simulink model "PSO_tunning_PID"  (R2017a)
settings: Solver=ode23s  StartTime=0.0  StopTime=10  RelTol=1000000
undefined symbols (not defined in the file or in its folder): kk
libraries: simulink x2
settings Model: Creator=abdul  LastModifiedBy=Dr. Javed
settings DataIOCC: SaveFormat=Array

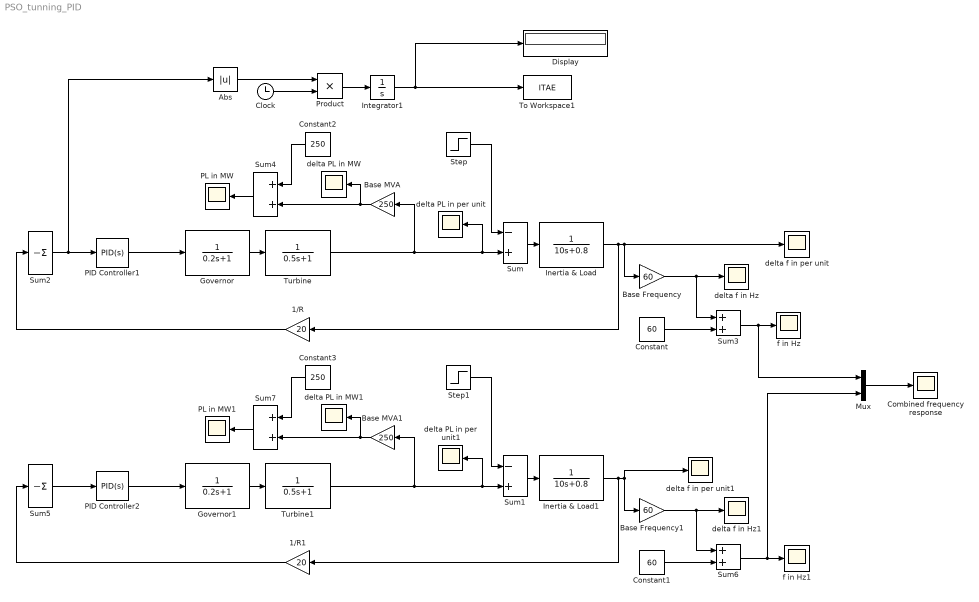
== system PSO_tunning_PID ==
  1/R : Gain  Gain=20
  1/R1 : Gain  Gain=20
  Abs : Abs
  Base Frequency : Gain  Gain=60
  Base Frequency1 : Gain  Gain=60
  Base MVA : Gain  Gain=250
  Base MVA1 : Gain  Gain=250
  Clock : Clock
  "Combined frequency response " : Scope
  Constant : Constant  Value=60
  Constant1 : Constant  Value=60
  Constant2 : Constant  Value=250
  Constant3 : Constant  Value=250
  Display : Display
      settings: Format=decimal (Stored Integer)
  Governor : TransferFcn  Denominator=[0.2 1]
  Governor1 : TransferFcn  Denominator=[0.2 1]
  Inertia & Load : TransferFcn  Denominator=[10 0.8]
  Inertia & Load1 : TransferFcn  Denominator=[10 0.8]
  Integrator1 : Integrator
  Mux : Mux  Inputs=2
  PID Controller1 : simulink/Continuous/PID Controller  Controller=PID  TimeDomain=Continuous-time  SampleTime=-1  IntegratorMethod=Forward Euler  FilterMethod=Forward Euler  Form=Parallel  UseFilter=on  ControllerParametersSource=internal  P=kk(1)  I=kk(2)  D=kk(3)  N=100  InitialConditionSource=internal  InitialConditionForIntegrator=0  InitialConditionForFilter=0  ExternalReset=none  LimitOutput=off  UpperSaturationLimit=inf  LowerSaturationLimit=-inf  LinearizeAsGain=on  AntiWindupMode=none  Kb=1  TrackingMode=off  Kt=1  PParamMin=[]  PParamMax=[]  IParamMin=[]  IParamMax=[]  DParamMin=[]  DParamMax=[]  NParamMin=[]  NParamMax=[]  KbParamMin=[]  KbParamMax=[]  KtParamMin=[]  KtParamMax=[]  POutMin=[]  POutMax=[]  IOutMin=[]  IOutMax=[]  DOutMin=[]  DOutMax=[]  NOutMin=[]  NOutMax=[]  KbOutMin=[]  KbOutMax=[]  KtOutMin=[]  KtOutMax=[]  IntegratorOutMin=[]  IntegratorOutMax=[]  FilterOutMin=[]  FilterOutMax=[]  SumOutMin=[]  SumOutMax=[]  SumI1OutMin=[]  SumI1OutMax=[]  SumI2OutMin=[]  SumI2OutMax=[]  SumI3OutMin=[]  SumI3OutMax=[]  SumDOutMin=[]  SumDOutMax=[]  SaturationOutMin=[]  SaturationOutMax=[]  IntegratorContinuousStateAttributes=''  IntegratorStateMustResolveToSignalObject=off  IntegratorRTWStateStorageClass=Auto  FilterContinuousStateAttributes=''  FilterStateMustResolveToSignalObject=off  FilterRTWStateStorageClass=Auto  DifferentiatorICPrevScaledInput=0  DifferentiatorOutMin=[]  DifferentiatorOutMax=[]  InitialConditionSetting=State (most efficient)
  PID Controller2 : simulink/Continuous/PID Controller  Controller=PID  TimeDomain=Continuous-time  SampleTime=-1  IntegratorMethod=Forward Euler  FilterMethod=Forward Euler  Form=Parallel  UseFilter=on  ControllerParametersSource=internal  P=2  I=1  D=1  N=100  InitialConditionSource=internal  InitialConditionForIntegrator=0  InitialConditionForFilter=0  ExternalReset=none  LimitOutput=off  UpperSaturationLimit=inf  LowerSaturationLimit=-inf  LinearizeAsGain=on  AntiWindupMode=none  Kb=1  TrackingMode=off  Kt=1  PParamMin=[]  PParamMax=[]  IParamMin=[]  IParamMax=[]  DParamMin=[]  DParamMax=[]  NParamMin=[]  NParamMax=[]  KbParamMin=[]  KbParamMax=[]  KtParamMin=[]  KtParamMax=[]  POutMin=[]  POutMax=[]  IOutMin=[]  IOutMax=[]  DOutMin=[]  DOutMax=[]  NOutMin=[]  NOutMax=[]  KbOutMin=[]  KbOutMax=[]  KtOutMin=[]  KtOutMax=[]  IntegratorOutMin=[]  IntegratorOutMax=[]  FilterOutMin=[]  FilterOutMax=[]  SumOutMin=[]  SumOutMax=[]  SumI1OutMin=[]  SumI1OutMax=[]  SumI2OutMin=[]  SumI2OutMax=[]  SumI3OutMin=[]  SumI3OutMax=[]  SumDOutMin=[]  SumDOutMax=[]  SaturationOutMin=[]  SaturationOutMax=[]  IntegratorContinuousStateAttributes=''  IntegratorStateMustResolveToSignalObject=off  IntegratorRTWStateStorageClass=Auto  FilterContinuousStateAttributes=''  FilterStateMustResolveToSignalObject=off  FilterRTWStateStorageClass=Auto  DifferentiatorICPrevScaledInput=0  DifferentiatorOutMin=[]  DifferentiatorOutMax=[]  InitialConditionSetting=State (most efficient)
  PL in MW : Scope
  PL in MW1 : Scope
  Product : Product
  Step : Step  Time=100  Before=0.2  After=0.2  SampleTime=0
  Step1 : Step  Time=100  Before=0.2  After=0.2  SampleTime=0
  Sum : Sum  Inputs=-+
  Sum1 : Sum  Inputs=-+
  Sum2 : Sum  Inputs=-
  Sum{3..4,6..7} (4 alike) : Sum
  Sum5 : Sum  Inputs=-
  To Workspace1 : ToWorkspace  VariableName=ITAE  SampleTime=-1
      settings: Save2DSignal=2-D array (concatenate along first dimension)
  Turbine : TransferFcn  Denominator=[0.5 1]
  Turbine1 : TransferFcn  Denominator=[0.5 1]
  delta PL in MW : Scope
  delta PL in MW1 : Scope
  delta PL in per unit : Scope
  delta PL in per unit1 : Scope
  delta f in Hz : Scope
  delta f in Hz1 : Scope
  delta f in per unit : Scope
  delta f in per unit1 : Scope
  f in Hz : Scope
  f in Hz1 : Scope
  wires:
  Sum3/1 -> Mux/1, f in Hz/1
  Constant/1 -> Sum3/2
  Inertia & Load/1 -> delta f in per unit/1, Base Frequency/1, 1/R/1
  1/R/1 -> Sum2/1
  Sum/1 -> Inertia & Load/1
  Governor/1 -> Turbine/1
  Base Frequency/1 -> delta f in Hz/1, Sum3/1
  Turbine/1 -> Base MVA/1, delta PL in per unit/1, Sum/2
  Base MVA/1 -> Sum4/2, delta PL in MW/1
  Sum4/1 -> PL in MW/1
  Step/1 -> Sum/1
  Constant2/1 -> Sum4/1
  PID Controller1/1 -> Governor/1
  Turbine1/1 -> Base MVA1/1, delta PL in per unit1/1, Sum1/2
  Step1/1 -> Sum1/1
  Sum7/1 -> PL in MW1/1
  Base MVA1/1 -> Sum7/2, delta PL in MW1/1
  Constant3/1 -> Sum7/1
  Sum1/1 -> Inertia & Load1/1
  Governor1/1 -> Turbine1/1
  Base Frequency1/1 -> delta f in Hz1/1, Sum6/1
  Sum6/1 -> Mux/2, f in Hz1/1
  Sum5/1 -> PID Controller2/1
  PID Controller2/1 -> Governor1/1
  1/R1/1 -> Sum5/1
  Inertia & Load1/1 -> delta f in per unit1/1, Base Frequency1/1, 1/R1/1
  Constant1/1 -> Sum6/2
  Mux/1 -> "Combined frequency response "/1
  Clock/1 -> Product/2
  Abs/1 -> Product/1
  Integrator1/1 -> To Workspace1/1, Display/1
  Sum2/1 -> Abs/1, PID Controller1/1
  Product/1 -> Integrator1/1
